simulink model "sampleModel54"  (R2021b)
settings: Solver=VariableStepAuto  StartTime=0.0  StopTime=10.0  RelTol=1e-3
libraries: simulink x4, slpidlib x2
settings Model: Creator=user  LastModifiedBy=user

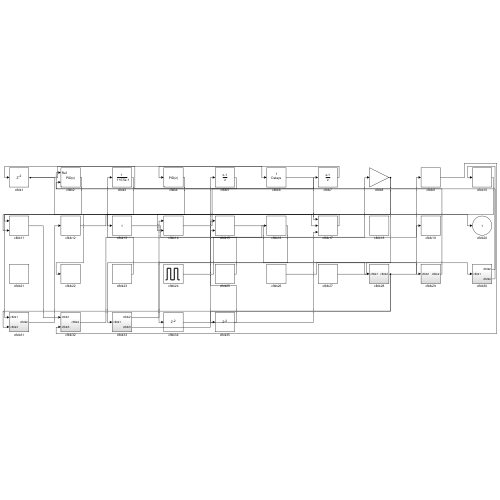
[thumbnail: Simulink's stored preview of the top-level diagram]
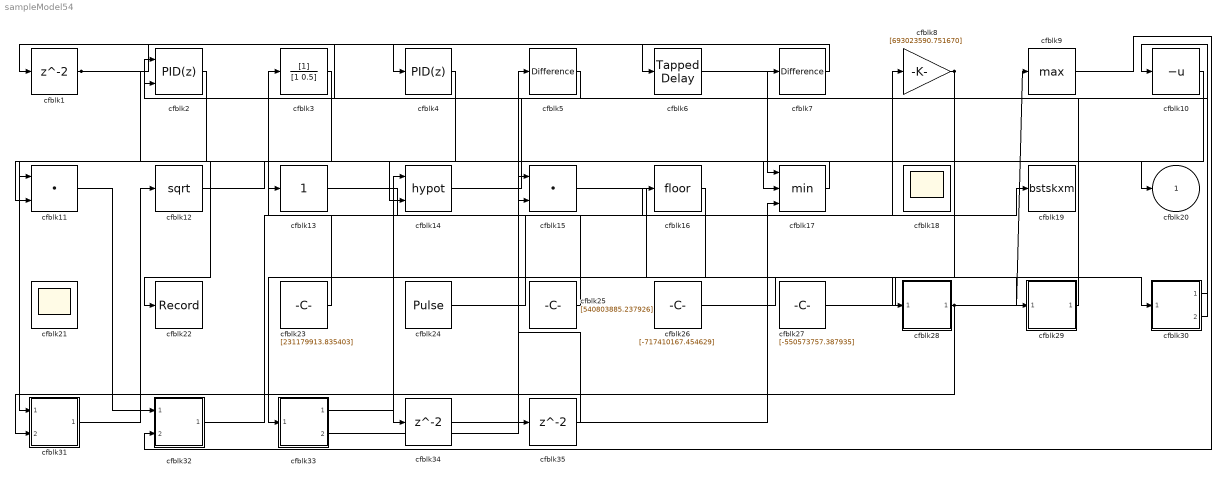
== system sampleModel54 ==
  cfblk1 : Delay  SampleTime=1
  cfblk10 : UnaryMinus
  cfblk11 : DotProduct  InputSameDT=on  OutDataTypeStr=Inherit: Inherit via internal rule
  cfblk12 : Sqrt  SaturateOnIntegerOverflow=on
  cfblk13 : simulink/Math Operations/Slider Gain  gain=1  low=0  high=2
  cfblk14 : Math  Operator=hypot  SaturateOnIntegerOverflow=on
  cfblk15 : DotProduct  InputSameDT=on  OutDataTypeStr=Inherit: Inherit via internal rule
  cfblk16 : Rounding
  cfblk17 : MinMax  Inputs=3
  cfblk18 : Scope
      settings: Floating=on
  cfblk19 : ToWorkspace  VariableName=bstskxm  SaveFormat=Timeseries  SampleTime=-1
  cfblk2 : slpidlib/PID Controller (2DOF)  Controller=PID  Form=Parallel  TimeDomain=Discrete-time  UseExternalTs=off  SampleTime=1  IntegratorMethod=Forward Euler  FilterMethod=Forward Euler  ControllerParametersSource=internal  P=1  I=1  D=0  UseFilter=on  N=100  b=1  c=1  TunerSelectOption=Transfer Function Based (PID Tuner App)  InitialConditionSource=internal  InitialConditionForIntegrator=0  InitialConditionForFilter=0  DifferentiatorICPrevScaledInput=0  ExternalReset=none  TrackingMode=off  Kt=1  LimitOutput=off  SatLimitsSource=internal  UpperSaturationLimit=inf  LowerSaturationLimit=-inf  LinearizeAsGain=off  AntiWindupMode=none  Kb=1  POutMin=[]  POutMax=[]  IOutMin=[]  IOutMax=[]  DOutMin=[]  DOutMax=[]  NOutMin=[]  NOutMax=[]  bOutMin=[]  bOutMax=[]  cOutMin=[]  cOutMax=[]  SumOutMin=[]  SumOutMax=[]  SaturationOutMin=[]  SaturationOutMax=[]  PParamMin=[]  PParamMax=[]  IParamMin=[]  IParamMax=[]  DParamMin=[]  DParamMax=[]  NParamMin=[]  NParamMax=[]  bParamMin=[]  bParamMax=[]  cParamMin=[]  cParamMax=[]  KbParamMin=[]  KbParamMax=[]  KtParamMin=[]  KtParamMax=[]  KbOutMin=[]  KbOutMax=[]  KtOutMin=[]  KtOutMax=[]  IntegratorOutMin=[]  IntegratorOutMax=[]  FilterOutMin=[]  FilterOutMax=[]  SumI1OutMin=[]  SumI1OutMax=[]  SumI2OutMin=[]  SumI2OutMax=[]  SumI3OutMin=[]  SumI3OutMax=[]  SumI4OutMin=[]  SumI4OutMax=[]  SumDOutMin=[]  SumDOutMax=[]  Sum1OutMin=[]  Sum1OutMax=[]  Sum2OutMin=[]  Sum2OutMax=[]  Sum3OutMin=[]  Sum3OutMax=[]  DifferentiatorOutMin=[]  DifferentiatorOutMax=[]  FilterDiffOutCoefMin=[]  FilterDiffOutCoefMax=[]  ReciprocalOutMin=[]  ReciprocalOutMax=[]  SumDenOutMin=[]  SumDenOutMax=[]  SumNumOutMin=[]  SumNumOutMax=[]  DivideOutMin=[]  DivideOutMax=[]  UdiffTsProdOutMin=[]  UdiffTsProdOutMax=[]  NTsProdOutMin=[]  NTsProdOutMax=[]  UintegralTsProdOutMin=[]  UintegralTsProdOutMax=[]  UngainTsProdOutMin=[]  UngainTsProdOutMax=[]  IntegratorContinuousStateAttributes=''  IntegratorStateMustResolveToSignalObject=off  IntegratorRTWStateStorageClass=Auto  FilterContinuousStateAttributes=''  FilterStateMustResolveToSignalObject=off  FilterRTWStateStorageClass=Auto  ParallelPVariant=InternalParameters  IdealPVariant=Disabled  IVariant=InternalParameters  DVariant=InternalParameters  bVariant=InternalParameters  cVariant=InternalParameters  IntegratorVariant=Discrete  SatVariant=Disabled  AWVariant=Passthrough  PCopyVariant=Disabled  TRVariant=Disabled  FdbkBlocksVariant=Forward  IdealPFdbkVariant=Disabled  SatFdbkVariant=Disabled  DerivativeFilterVariant=ForwardEulerFilter  NVariant=InternalParameters  NCopyVariant=Disabled  FilterICVariant=InternalICsFilter  IntegratorICVariant=InternalICs  ExternalResetVariant=Disabled  TRSumVariant=Passthrough  SumFdbkVariant=Disabled  SumVariant=Sum_PID  TsampFilterVariant=InternalTs  TsampNgainVariant=Passthrough  TsampIntegralVariant=Passthrough  ExternalSaturationOutDataTypeStr=Inherit: Same as second input
      settings: SourceProductBaseCode=SL
  cfblk21 : Scope
      settings: Floating=on
  cfblk22 : Record  FileSettingsInternal="{\"entries\":[{\"content\":{\"excelSettings\":{\"content\":{},\"type\":\"Streamout.ExcelSettings\"}},\"type\":\"Streamout.FileSettingStorage\",\"uuid\":\"22d2adfe-9bd1-4db2-90bf-b38fd4f97270\"}],\"packageUris\":[\"http://schema.mathworks.com/mf0/streamout_blocks/R2020a\"],\"version\":\"1.0\"}"  SignalsInternal="{\"entries\":[{\"content\":{\"signals\":[{\"content\":{\"blockPath\":[\"sampleModel54/cfblk22\"],\"channel\":[],\"dimensions\":[1],\"domain\":\"sampleModel54/cfblk22\",\"lineColor\":\"#77ac30\",\"plots\":[1],\"port\":1,\"sid\":[\"\"],\"signalID\":2114,\"signalName\":\"cfblk4\"},\"type\":\"RecordBlkView.Signal\",\"uuid\":\"4f44760a-0729-4a1c-9f22-ab4dd7369289\"}]},\"type\":\"RecordBlkView.InputSignals\",\"uuid\":\"fda242ae-869b-431d-8caf-527f3e83d201\"}],\"packageUris\":[\"http://schema.mathworks.com/mf0/streamout_blocks/R2020a\"],\"version\":\"1.0\"}"  VisualizationBindings="{\"sparklinesplugin\":{\"info\":[{\"bindingParametersList\":[],\"subplotID\":1}]}}"
  cfblk23 : Constant  Value=[231179913.835403]  SampleTime=1
  cfblk24 : DiscretePulseGenerator  PulseType=Time based  Amplitude=[670500118.444290]  Period=[44677237.293250]  PulseWidth=5  PhaseDelay=[9.000000]
  cfblk25 : Constant  Value=[540803885.237926]  SampleTime=1
  cfblk26 : Constant  Value=[-717410167.454629]  SampleTime=1
  cfblk27 : Constant  Value=[-550573757.387935]  SampleTime=1
  cfblk28 : Subsystem
  cfblk29 : Subsystem
  cfblk3 : DiscreteFilter  SampleTime=1
  cfblk30 : Subsystem
  cfblk31 : Subsystem
  cfblk32 : Subsystem
  cfblk33 : Subsystem
  cfblk34 : Delay  SampleTime=1
  cfblk35 : Delay  SampleTime=1
  cfblk4 : slpidlib/PID Controller  Controller=PID  Form=Parallel  TimeDomain=Discrete-time  UseExternalTs=off  SampleTime=1  IntegratorMethod=Forward Euler  FilterMethod=Forward Euler  ControllerParametersSource=internal  P=1  I=1  D=0  UseFilter=on  N=100  TunerSelectOption=Transfer Function Based (PID Tuner App)  InitialConditionSource=internal  InitialConditionForIntegrator=0  InitialConditionForFilter=0  DifferentiatorICPrevScaledInput=0  ExternalReset=none  TrackingMode=off  Kt=1  LimitOutput=off  SatLimitsSource=internal  UpperSaturationLimit=inf  LowerSaturationLimit=-inf  LinearizeAsGain=off  AntiWindupMode=none  Kb=1  POutMin=[]  POutMax=[]  IOutMin=[]  IOutMax=[]  DOutMin=[]  DOutMax=[]  NOutMin=[]  NOutMax=[]  SumOutMin=[]  SumOutMax=[]  SaturationOutMin=[]  SaturationOutMax=[]  PParamMin=[]  PParamMax=[]  IParamMin=[]  IParamMax=[]  DParamMin=[]  DParamMax=[]  NParamMin=[]  NParamMax=[]  KbParamMin=[]  KbParamMax=[]  KtParamMin=[]  KtParamMax=[]  KbOutMin=[]  KbOutMax=[]  KtOutMin=[]  KtOutMax=[]  IntegratorOutMin=[]  IntegratorOutMax=[]  FilterOutMin=[]  FilterOutMax=[]  SumI1OutMin=[]  SumI1OutMax=[]  SumI2OutMin=[]  SumI2OutMax=[]  SumI3OutMin=[]  SumI3OutMax=[]  SumI4OutMin=[]  SumI4OutMax=[]  SumDOutMin=[]  SumDOutMax=[]  DifferentiatorOutMin=[]  DifferentiatorOutMax=[]  FilterDiffOutCoefMin=[]  FilterDiffOutCoefMax=[]  ReciprocalOutMin=[]  ReciprocalOutMax=[]  SumDenOutMin=[]  SumDenOutMax=[]  SumNumOutMin=[]  SumNumOutMax=[]  DivideOutMin=[]  DivideOutMax=[]  UdiffTsProdOutMin=[]  UdiffTsProdOutMax=[]  NTsProdOutMin=[]  NTsProdOutMax=[]  UintegralTsProdOutMin=[]  UintegralTsProdOutMax=[]  UngainTsProdOutMin=[]  UngainTsProdOutMax=[]  IntegratorContinuousStateAttributes=''  IntegratorStateMustResolveToSignalObject=off  IntegratorRTWStateStorageClass=Auto  FilterContinuousStateAttributes=''  FilterStateMustResolveToSignalObject=off  FilterRTWStateStorageClass=Auto  ParallelPVariant=InternalParameters  IdealPVariant=Disabled  IVariant=InternalParameters  DVariant=InternalParameters  IntegratorVariant=Discrete  SatVariant=Disabled  AWVariant=Passthrough  PCopyVariant=Disabled  TRVariant=Disabled  FdbkBlocksVariant=Forward  IdealPFdbkVariant=Disabled  SatFdbkVariant=Disabled  DerivativeFilterVariant=ForwardEulerFilter  NVariant=InternalParameters  NCopyVariant=Disabled  FilterICVariant=InternalICsFilter  IntegratorICVariant=InternalICs  ExternalResetVariant=Disabled  TRSumVariant=Passthrough  SumFdbkVariant=Disabled  SumVariant=Sum_PID  TsampFilterVariant=InternalTs  TsampNgainVariant=Passthrough  TsampIntegralVariant=Passthrough  ExternalSaturationOutDataTypeStr=Inherit: Same as second input
  cfblk5 : simulink/Discrete/Difference  ICPrevInput=0.0  OutMin=[]  OutMax=[]  OutDataTypeStr=Inherit: Inherit via back propagation  OutDataType=fixdt(1, 16)  OutScaling=2^-10  DoSatur=off
  cfblk6 : simulink/Discrete/Tapped Delay  vinit=0.0  samptime=-1  NumDelays=1  DelayOrder=Oldest  includeCurrent=off
  cfblk7 : simulink/Discrete/Difference  ICPrevInput=0.0  OutMin=[]  OutMax=[]  OutDataTypeStr=Inherit: Inherit via back propagation  OutDataType=fixdt(1, 16)  OutScaling=2^-10  DoSatur=off
  cfblk8 : Gain  Gain=[693023590.751670]
  cfblk9 : MinMax  Function=max
  cfblk20 : Outport
  wires:
  cfblk7/1 -> cfblk4/1
  cfblk2/1 -> cfblk31/1(cfblk1)
  cfblk23/1 -> cfblk3/1
  cfblk5/1 -> cfblk1/1
  cfblk17/1 -> cfblk13/1
  cfblk13/1 -> cfblk8/1
  cfblk11/1 -> cfblk32/1(cfblk1)
  cfblk6/1 -> cfblk17/1
  cfblk31/1(cfblk2) -> cfblk12/1
  cfblk16/1 -> cfblk33/1(cfblk1)
  cfblk27/1 -> cfblk30/1(cfblk1)
  cfblk1/1 -> cfblk6/1, cfblk20/1
  cfblk15/1 -> cfblk28/1(cfblk1)
  cfblk28/1(cfblk2) -> cfblk9/1, cfblk31/2(cfblk3), cfblk35/1
  cfblk32/1(cfblk2) -> cfblk19/1
  cfblk10/1 -> cfblk11/1
  cfblk3/1 -> cfblk11/2
  cfblk30/1(cfblk2) -> cfblk10/1
  cfblk25/1 -> cfblk5/1
  cfblk30/2(cfblk4) -> cfblk2/1
  cfblk9/1 -> cfblk32/2(cfblk3)
  cfblk33/1(cfblk2) -> cfblk14/1
  cfblk26/1 -> cfblk29/1(cfblk1)
  cfblk24/1 -> cfblk16/1
  cfblk12/1 -> cfblk17/2
  cfblk4/1 -> cfblk22/1
  cfblk29/1(cfblk2) -> cfblk2/2
  cfblk8/1 -> cfblk14/2, cfblk34/1
  cfblk14/1 -> cfblk7/1
  cfblk33/2(cfblk5) -> cfblk15/1
  cfblk34/1 -> cfblk17/3
  cfblk35/1 -> cfblk15/2

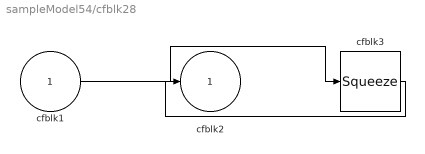
== system sampleModel54/cfblk28 ==
  cfblk1 : Inport
  cfblk3 : Squeeze
  cfblk2 : Outport
  wires:
  cfblk1/1 -> cfblk3/1
  cfblk3/1 -> cfblk2/1

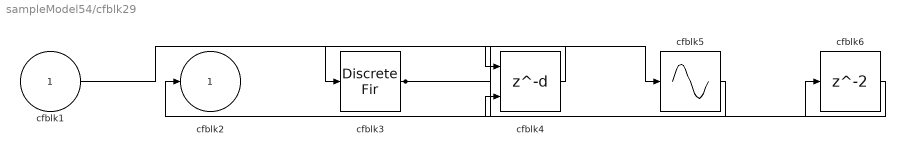
== system sampleModel54/cfblk29 ==
  cfblk1 : Inport
  cfblk3 : DiscreteFir  SampleTime=1
  cfblk4 : Delay  DelayLengthSource=Input port  SampleTime=1
      settings: InputPortMap=u0,p1
  cfblk5 : Sin  TimeSource=Use external signal  SampleTime=0
  cfblk6 : Delay  SampleTime=1
  cfblk2 : Outport
  wires:
  cfblk3/1 -> cfblk5/1, cfblk6/1
  cfblk5/1 -> cfblk2/1
  cfblk1/1 -> cfblk4/1
  cfblk4/1 -> cfblk3/1
  cfblk6/1 -> cfblk4/2

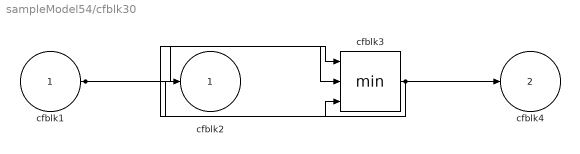
== system sampleModel54/cfblk30 ==
  cfblk1 : Inport
  cfblk3 : MinMax  Inputs=3
  cfblk2 : Outport
  cfblk4 : Outport  Port=2
  wires:
  cfblk1/1 -> cfblk3/1, cfblk3/2, cfblk3/3
  cfblk3/1 -> cfblk2/1, cfblk4/1

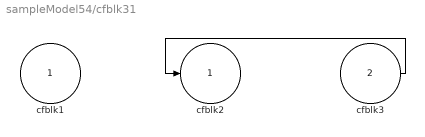
== system sampleModel54/cfblk31 ==
  cfblk1 : Inport
  cfblk3 : Inport  Port=2
  cfblk2 : Outport
  wires:
  cfblk3/1 -> cfblk2/1

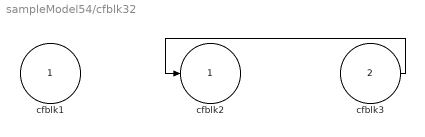
== system sampleModel54/cfblk32 ==
  cfblk1 : Inport
  cfblk3 : Inport  Port=2
  cfblk2 : Outport
  wires:
  cfblk3/1 -> cfblk2/1

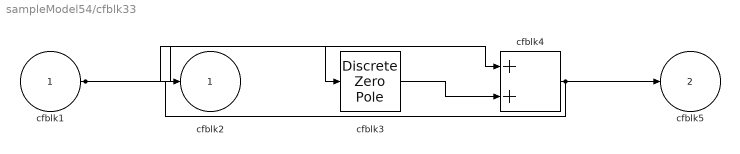
== system sampleModel54/cfblk33 ==
  cfblk1 : Inport
  cfblk3 : DiscreteZeroPole  Poles=[0 0.5]  Gain=1
  cfblk4 : Sum
  cfblk2 : Outport
  cfblk5 : Outport  Port=2
  wires:
  cfblk1/1 -> cfblk4/1, cfblk3/1
  cfblk3/1 -> cfblk4/2
  cfblk4/1 -> cfblk2/1, cfblk5/1
